simulink model "drivecycle"  (R2024b)
settings: Solver=VariableStepAuto  StartTime=0.0  StopTime=1800  RelTol=1e-3
undefined symbols (not defined in the file or in its folder): Ion, Lithium
libraries: nesl_utility x6, sdl_lib x2, spsBatteryLib x1, autolibmappedmotor x1, fl_lib x1, slpidlib x1, sps_lib x1
settings Model: SimulationMode=accelerator  Creator=srich  LastModifiedBy=srich
settings DataIOCC: LoggingToFile=on

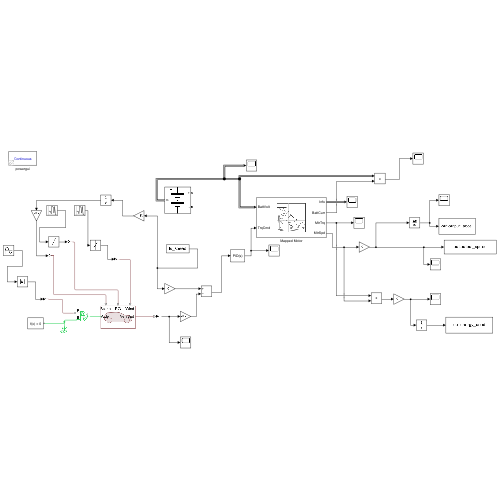
[thumbnail: Simulink's stored preview of the top-level diagram]
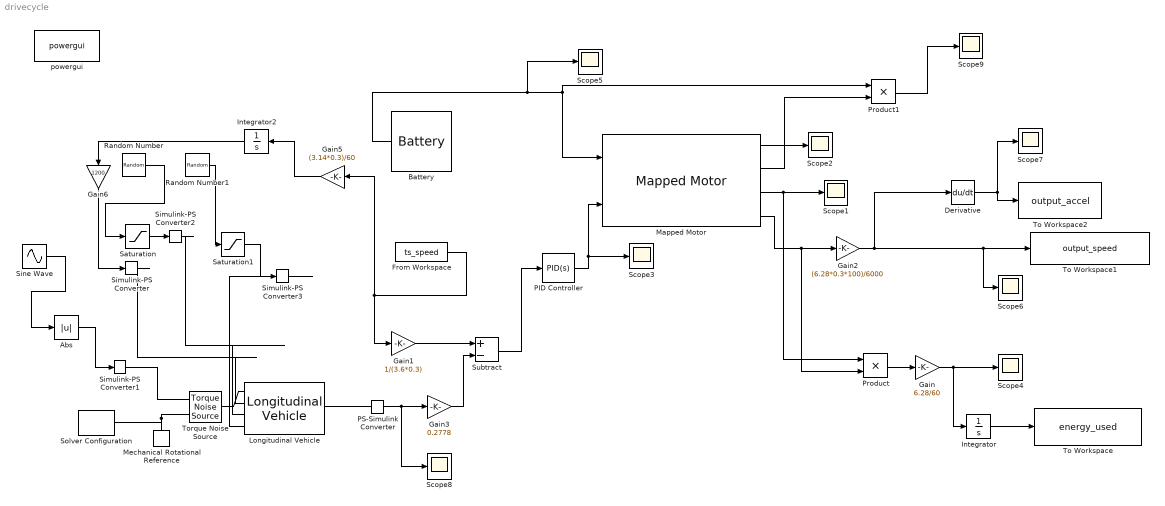
== system drivecycle ==
  Abs : Abs  SaturateOnIntegerOverflow=off
  Battery : spsBatteryLib/Battery  BatType=Lithium-Ion  NomV=360  NomQ=120  SOC=100  Batt_Tr=1e-3  PresetModel=on  MaxQ=120  MinV=270  FullV=419.0354  Dis_rate=52.1739  R=0.03  Normal_OP=108.5217  expZone="[388.9389      5.895652]"
  Derivative : Derivative
  From Workspace : FromWorkspace  VariableName=ts_speed  SampleTime=-1
  Gain : Gain  Gain=6.28/60
  Gain1 : Gain  Gain=1/(3.6*0.3)
  Gain2 : Gain  Gain=(6.28*0.3*100)/6000
  Gain3 : Gain  Gain=0.2778
  Gain5 : Gain  Gain=(3.14*0.3)/60
  Gain6 : Gain  Gain=1200
  Integrator : Integrator
  Integrator2 : Integrator
  Longitudinal Vehicle : sdl_lib/Tires & Vehicles/Longitudinal Vehicle  vehParamType=sdl.enum.VehicleParameterizationType.Regular  M_vehicle=1200 kg  R_tireroll=0.3 m  C_tireroll=0.015  C_airdrag=0.29  A_front=2.2 m^2  A_rl=120 N  B_rl=1.8 N*s/m  C_rl=0.389 N*s^2/m^2  g=9.81 m/s^2  V_1=0.3 m/s  w_1=0.01 rad/s  ShowBrakeIn=true  ShowSlopeIn=true  SlopeInputType=sdl.enum.VehicleLongitudinalRoadSlopeInputType.GradePercent  ShowWindIn=true  ShowGOut=false  air_density=1.184 kg/m^3  V_x_specify=off  V_x_priority=High  V_x=0 m/s  V_x_nominal_specify=off  V_x_nominal_value=1  V_x_nominal_unit=m/s  trq_specify=off  trq_priority=None  trq=0 N*m  trq_nominal_specify=off  trq_nominal_value=1  trq_nominal_unit=N*m  w_specify=off  w_priority=None  w=0 rad/s  w_nominal_specify=off  w_nominal_value=1  w_nominal_unit=rad/s
      settings: InternalSimscapePortConfiguration="{\"Bottom\":[],\"Left\":[{\"id\":\"Axle\",\"label\":\"Axle\",\"type\":\"foundation.mechanical.rotational.rotational\"}],\"Right\":[{\"id\":\"v_out\",\"label\":\"VehSpd\",\"type\":\"output\"}],\"Top\":[{\"id\":\"brkF\",\"label\":\"Brake\",\"type\":\"input\"},{\"id\":\"grade_pct\",\"label\":\"PG\",\"type\":\"input\"},{\"id\":\"V_wind\",\"label\":\"Wind\",\"type\":\"input\"}]}"
  Mapped Motor : autolibmappedmotor/Mapped Motor  w_Tmax_bp_ext=w_Tmax_bp  Tmax_w_V_ext=Tmax_w_V  w_Tmin_bp_ext=w_Tmin_bp  Tmin_w_V_ext=Tmin_w_V  port_config=Torque  param_by=Tabulated torque-speed envelope  w_t=[ 0 375 750 800 ]  T_t=[0.09 0.08 0.07 0]  torque_max=.1  power_max=30  SpreadsheetTqLimitsFileName=MotorCalibrationImportData.xlsx  Tmax_w_V=[0.09 0.09 0.09;0.08 0.08 0.08;0.07 0.07 0.07;0 0 0]  w_Tmax_bp=[ 0 375 750 800 ]  V_Tmax_bp=[500 750 900]  Tmin_w_V=[-0.09 -0.09 -0.09;-0.08 -0.08 -0.08;-0.07 -0.07 -0.07;0 0 0]  w_Tmin_bp=[ 0 375 750 800 ]  V_Tmin_bp=[500 750 900]  Tc=0.02  param_loss=Single efficiency measurement  SpreadsheetLossFileName=MotorCalibrationImportData.xlsx  SpreadsheetEffFileName=MotorCalibrationImportData.xlsx  eff=100  w_eff=375  T_eff=0.08  Piron=0  Pbase=0  w_eff_bp=[-800 -400 0 400 800]  T_eff_bp=[0 0.03 0.06 0.09]  Temp_eff_bp=[233.15 293.15 373.15]  V_eff_bp=[500 700 900]  losses_table=[1.49 1.67 2.21 3.10; 0.42 0.69 1.14 2.03; 0.06 0.24 0.78 1.68; 0.42 0.69 1.14 2.03; 1.49 1.67 2.21 3.10]  losses_table_3d=cat(3,[1.49 1.67 2.21 3.10; 0.42 0.69 1.14 2.03; 0.06 0.24 0.78 1.68; 0.42 0.69 1.14 2.03; 1.49 1.67 2.21 3.10],[1.49 1.67 2.21 3.10; 0.42 0.69 1.14 2.03; 0.06 0.24 0.78 1.68; 0.42 0.69 1.14 2.03; 1.49 1.67 2.21 3.10],[1.49 1.67 2.21 3.10; 0.42 0.69 1.14 2.03; 0.06 0.24 0.78 1.68; 0.42 0.69 1.14 2.03; 1.49 1.67 2.21 3.10])  losses_table_4d=cat(4,cat(3,[1.5645 0.441 0.063 0.441 1.5645;1.7535 0.7245 0.252 0.7245 1.7535;2.3205 1.197 0.819 1.197 2.3205;3.255 2.1315 1.764 2.1315 3.255],[1.5645 0.441 0.063 0.441 1.5645;1.7535 0.7245 0.252 0.7245 1.7535;2.3205 1.197 0.819 1.197 2.3205;3.255 2.1315 1.764 2.1315 3.255],[1.5645 0.441 0.063 0.441 1.5645;1.7535 0.7245 0.252 0.7245 1.7535;2.3205 1.197 0.819 1.197 2.3205;3.255 2.1315 1.764 2.1315 3.255]),cat(3,[1.49 0.42 0.06 0.42 1.49;1.67 0.69 0.24 0.69 1.67;2.21 1.14 0.78 1.14 2.21;3.1 2.03 1.68 2.03 3.1],[1.49 0.42 0.06 0.42 1.49;1.67 0.69 0.24 0.69 1.67;2.21 1.14 0.78 1.14 2.21;3.1 2.03 1.68 2.03 3.1],[1.49 0.42 0.06 0.42 1.49;1.67 0.69 0.24 0.69 1.67;2.21 1.14 0.78 1.14 2.21;3.1 2.03 1.68 2.03 3.1]),cat(3,[1.5347 0.4326 0.0618 0.4326 1.5347;1.7201 0.7107 0.2472 0.7107 1.7201;2.2763 1.1742 0.8034 1.1742 2.2763;3.193 2.0909 1.7304 2.0909 3.193],[1.5347 0.4326 0.0618 0.4326 1.5347;1.7201 0.7107 0.2472 0.7107 1.7201;2.2763 1.1742 0.8034 1.1742 2.2763;3.193 2.0909 1.7304 2.0909 3.193],[1.5347 0.4326 0.0618 0.4326 1.5347;1.7201 0.7107 0.2472 0.7107 1.7201;2.2763 1.1742 0.8034 1.1742 2.2763;3.193 2.0909 1.7304 2.0909 3.193]))  efficiency_table=[95 95 95 95; 95 95 95 95; 95 95 95 95; 95 95 95 95; 95 95 95 95]  efficiency_table_3d=cat(3,[95 95 95 95; 95 95 95 95; 95 95 95 95; 95 95 95 95; 95 95 95 95],[95 95 95 95; 95 95 95 95; 95 95 95 95; 95 95 95 95; 95 95 95 95],[95 95 95 95; 95 95 95 95; 95 95 95 95; 95 95 95 95; 95 95 95 95])  efficiency_table_4d=cat(4,cat(3,90*ones(5,4)',90*ones(5,4)',90*ones(5,4)'),cat(3,95*ones(5,4)',95*ones(5,4)',95*ones(5,4)'),cat(3,92*ones(5,4)',92*ones(5,4)',92*ones(5,4)'))  J=5e-6  b=1e-5  omega_o=0  T_t_extended=[0 0.07 0.08 0.09 0.08 0.07 0]  w_t_extended=[-800 -750 -375 0 375 750 800]  KLossIron=0  KLossCopper=0  x_w_eff_vec=[-8000 -4000 0 4000 8000]  x_T_eff_vec=[-0.09 -0.06 -0.03 0 0.03 0.06 0.09]  x_tmp_eff_vec=[-0.09 -0.06 -0.03 0 0.03 0.06 0.09]  x_V_eff_vec=[500 700 900]  x_losses_mat=[3.1 2.21 1.67 1.49 1.67 2.21 3.1;2.03 1.14 0.69 0.42 0.69 1.14 2.03;1.68 0.78 0.24 0.06 0.24 0.78 1.68;2.03 1.14 0.69 0.42 0.69 1.14 2.03;3.1 2.21 1.67 1.49 1.67 2.21 3.1]  x_losses_mat_3d=[37.8947368421052 25.2631578947368 12.6315789473684 0 12 24 36;18.9473684210526 12.6315789473684 6.3157894736842 0 5.99999999999999 12 18;0 0 0 0 0 0 0;18 12 5.99999999999999 0 6.3157894736842 12.6315789473684 18.9473684210526;36 24 12 0 12.6315789473684 25.2631578947368 37.8947368421052]  x_losses_mat_4d=cat(4,cat(3,[1.5645 0.441 0.063 0.441 1.5645;1.7535 0.7245 0.252 0.7245 1.7535;2.3205 1.197 0.819 1.197 2.3205;3.255 2.1315 1.764 2.1315 3.255],[1.5645 0.441 0.063 0.441 1.5645;1.7535 0.7245 0.252 0.7245 1.7535;2.3205 1.197 0.819 1.197 2.3205;3.255 2.1315 1.764 2.1315 3.255],[1.5645 0.441 0.063 0.441 1.5645;1.7535 0.7245 0.252 0.7245 1.7535;2.3205 1.197 0.819 1.197 2.3205;3.255 2.1315 1.764 2.1315 3.255]),cat(3,[1.49 0.42 0.06 0.42 1.49;1.67 0.69 0.24 0.69 1.67;2.21 1.14 0.78 1.14 2.21;3.1 2.03 1.68 2.03 3.1],[1.49 0.42 0.06 0.42 1.49;1.67 0.69 0.24 0.69 1.67;2.21 1.14 0.78 1.14 2.21;3.1 2.03 1.68 2.03 3.1],[1.49 0.42 0.06 0.42 1.49;1.67 0.69 0.24 0.69 1.67;2.21 1.14 0.78 1.14 2.21;3.1 2.03 1.68 2.03 3.1]),cat(3,[1.5347 0.4326 0.0618 0.4326 1.5347;1.7201 0.7107 0.2472 0.7107 1.7201;2.2763 1.1742 0.8034 1.1742 2.2763;3.193 2.0909 1.7304 2.0909 3.193],[1.5347 0.4326 0.0618 0.4326 1.5347;1.7201 0.7107 0.2472 0.7107 1.7201;2.2763 1.1742 0.8034 1.1742 2.2763;3.193 2.0909 1.7304 2.0909 3.193],[1.5347 0.4326 0.0618 0.4326 1.5347;1.7201 0.7107 0.2472 0.7107 1.7201;2.2763 1.1742 0.8034 1.1742 2.2763;3.193 2.0909 1.7304 2.0909 3.193]))  CalLossMapData={}  CalLossWithTempMapData={}  aMode=1  RefBlkName='autolibmappedmotor/Mapped Motor'
      settings: LibrarySourceBlock=autolibemachines/Mapped Motor
  Mechanical Rotational Reference : fl_lib/Mechanical/Rotational Elements/Mechanical Rotational Reference
  PID Controller : slpidlib/PID Controller  Controller=PID  Form=Parallel  TimeDomain=Continuous-time  UseExternalTs=off  SampleTime=-1  IntegratorMethod=Forward Euler  FilterMethod=Forward Euler  ControllerParametersSource=internal  P=1  I=0.1  UseKiTs=off  D=0.01  UseExternalDerivativeSource=off  N=1  UseFilter=on  TunerSelectOption=Transfer Function Based (PID Tuner App)  InitialConditionSource=internal  InitialConditionForIntegrator=0  InitialConditionForFilter=0  DifferentiatorICPrevScaledInput=0  ExternalReset=none  TrackingMode=off  Kt=1  LimitOutput=off  SatLimitsSource=internal  UpperSaturationLimit=inf  LowerSaturationLimit=-inf  LinearizeAsGain=on  AntiWindupMode=none  Kb=1  LimitIntegrator=off  UpperIntegratorSaturationLimit=inf  LowerIntegratorSaturationLimit=-inf  POutMin=[]  POutMax=[]  IOutMin=[]  IOutMax=[]  DOutMin=[]  DOutMax=[]  NOutMin=[]  NOutMax=[]  SumOutMin=[]  SumOutMax=[]  SaturationOutMin=[]  SaturationOutMax=[]  PParamMin=[]  PParamMax=[]  IParamMin=[]  IParamMax=[]  DParamMin=[]  DParamMax=[]  NParamMin=[]  NParamMax=[]  KbParamMin=[]  KbParamMax=[]  KtParamMin=[]  KtParamMax=[]  KbOutMin=[]  KbOutMax=[]  KtOutMin=[]  KtOutMax=[]  IntegratorOutMin=[]  IntegratorOutMax=[]  FilterOutMin=[]  FilterOutMax=[]  SumI1OutMin=[]  SumI1OutMax=[]  SumI2OutMin=[]  SumI2OutMax=[]  SumI3OutMin=[]  SumI3OutMax=[]  SumI4OutMin=[]  SumI4OutMax=[]  SumDOutMin=[]  SumDOutMax=[]  DifferentiatorOutMin=[]  DifferentiatorOutMax=[]  FilterDiffOutCoefMin=[]  FilterDiffOutCoefMax=[]  ReciprocalOutMin=[]  ReciprocalOutMax=[]  SumDenOutMin=[]  SumDenOutMax=[]  SumNumOutMin=[]  SumNumOutMax=[]  DivideOutMin=[]  DivideOutMax=[]  UdiffTsProdOutMin=[]  UdiffTsProdOutMax=[]  NTsProdOutMin=[]  NTsProdOutMax=[]  UintegralTsProdOutMin=[]  UintegralTsProdOutMax=[]  UngainTsProdOutMin=[]  UngainTsProdOutMax=[]  ClampingZeroOutDataTypeStr=Inherit: Inherit via back propagation  ClampingZeroOutMin=[]  ClampingZeroOutMax=[]  FilterDenConstantOutDataTypeStr=Inherit: Inherit via back propagation  FilterDenConstantOutMin=[]  FilterDenConstantOutMax=[]  PCopyOutDataTypeStr=Inherit: Inherit via back propagation  PCopyOutMin=[]  PCopyOutMax=[]  NCopyOutDataTypeStr=Inherit: Inherit via back propagation  NCopyOutMin=[]  NCopyOutMax=[]  IntegratorContinuousStateAttributes=''  IntegratorStateMustResolveToSignalObject=off  IntegratorRTWStateStorageClass=Auto  FilterContinuousStateAttributes=''  FilterStateMustResolveToSignalObject=off  FilterRTWStateStorageClass=Auto  ParallelPVariant=InternalParameters  IdealPVariant=Disabled  IVariant=InternalParameters  DVariant=InternalParameters  IntegratorVariant=Continuous  SatVariant=Disabled  AWVariant=Passthrough  PCopyVariant=Disabled  TRVariant=Disabled  FdbkBlocksVariant=Forward  IdealPFdbkVariant=Disabled  SatFdbkVariant=Disabled  DerivativeFilterVariant=ContFilter  NVariant=InternalParameters  NCopyVariant=Disabled  FilterICVariant=InternalICsFilter  IntegratorICVariant=InternalICs  ExternalResetVariant=Disabled  TRSumVariant=Passthrough  SumFdbkVariant=Disabled  SumVariant=Sum_PID  TsampFilterVariant=InternalTs  TsampNgainVariant=Passthrough  TsampIntegralVariant=Disabled_SignalSpec  ExternalSaturationOutDataTypeStr=Inherit: Same as second input  DerivativeSourceVariant=ErrorSignal  PreIntVariant=InternalPreInt
  PS-Simulink Converter : nesl_utility/PS-Simulink Converter  PhysicalDomain=network_engine_domain  SubClassName=ps_output  LeftPortType=input  RightPortType=output  PseudoPeriodic=off  Frequencies=[]  VectorFormat=inherit  Unit=inherit  AffineConversion=off
  Product : Product
  Product1 : Product
  Random Number : RandomNumber  Mean=6.5  Variance=0.5625  SampleTime=0.01
  Random Number1 : RandomNumber  Mean=7.5  Variance=0.5625  SampleTime=0.1
  Saturation : Saturate  UpperLimit=8  LowerLimit=5
  Saturation1 : Saturate  UpperLimit=10  LowerLimit=5
  Scope{1..9} (9 alike) : Scope
  Simulink-PS Converter{,1..3} (4 alike) : nesl_utility/Simulink-PS Converter  PhysicalDomain=network_engine_domain  SubClassName=ps_input  LeftPortType=input  RightPortType=output  PseudoPeriodic=off  Frequencies=[]  NoiseDistribution=none  NoiseParameters=[]  Unit=1  AffineConversion=off  FilteringAndDerivatives=provide  SimscapeFilterOrder=1  InputFilterTimeConstant=0.001  UdotUserProvided=0
  Sine Wave : Sin  Amplitude=5  Bias=5  Frequency=10  SampleTime=0
  Solver Configuration : nesl_utility/Solver Configuration  PhysicalDomain=network_engine_domain  SubClassName=solver  LeftPortType=input  RightPortType=generic  Tones=[]  Harmonics=[]  SimulateNoise=off  Profile=off  UseLocalSampling=off  EnableSwitchedLinearOptims=on  FrequencyDomain=off  UseCCode=off  RelTol=0.001  AbsTol=0.001  MinStep=1e-09  ToWorkspace=off  RevertToSquareIcSolve=off  NumHomotopyIterations=100  PhasorMode=off  PhasorModeNumHarmonics=1  ConsistencySolver=NEWTON_XTOL_AFTER_FTOL  IndexReductionMethod=DerivativeReplacement  DoDC=off  ResidualTolerance=1e-09  ConsistencyTolSource=GLOBAL  ConsistencyAbsTol=0.001  ConsistencyRelTol=0.001  ConsistencyTolFactor=0.001  UseLocalSolver=off  LocalSolverChoice=NE_BACKWARD_EULER_ADVANCER  ResolveIndetEquations=on  FunctionEvalNumThread=1  LocalSolverSampleTime=0.001  DoFixedCost=off  MaxNonlinIter=3  MaxModeIter=2  ComputeImpulses=off  ImpulseIterations=2  LinearAlgebra=auto  LinearAlgebraNumThread=0  EquationFormulation=NE_TIME_EF  DelaysMemoryBudget=1024  AutomaticFiltering=on  FilteringTimeConstant=0.001  PartitionStorageMethod=AS_NEEDED  PartitionMemoryBudget=1024  PartitionMethod=ROBUST  MultibodyUseLocalSolver=off  MultibodyLocalSolverChoice=ODE1  MultibodyLocalSolverSampleTime=0.001
  Subtract : Sum  Inputs=+-
  To Workspace : ToWorkspace  VariableName=energy_used  SaveFormat=Timeseries
  To Workspace1 : ToWorkspace  VariableName=output_speed  SaveFormat=Timeseries
  To Workspace2 : ToWorkspace  VariableName=output_accel  SaveFormat=Timeseries
  Torque Noise Source : sdl_lib/Sources/Torque Noise Source  sample_time=1e-3 s  repeatability=sdl.enum.seedInitialization.NotRepeatable  user_seed=0  auto_seed=3890346746
      settings: InternalSimscapePortConfiguration="{\"Bottom\":[],\"Left\":[{\"id\":\"PSD\",\"label\":\"P\",\"type\":\"input\"},{\"id\":\"B\",\"label\":\"B\",\"type\":\"foundation.mechanical.rotational.rotational\"}],\"Right\":[{\"id\":\"F\",\"label\":\"F\",\"type\":\"foundation.mechanical.rotational.rotational\"}],\"Top\":[]}"
  powergui : sps_lib/powergui  Priority=1  SimulationMode=Continuous  SampleTime=1800  frequency=60  Iterations=50  frequencyindice=0  Pbase=100e6  ErrMax=1e-4  UnitsV=kV  UnitsW=MW  buscounter=0  FunctionMessages=off  echomessages=off  EnableUseOfTLC=off  CurrentSourceSwitches=off  DisableSnubberDevices=off  DisableRonSwitches=off  DisableVfSwitches=off  DisplayEquations=off  AutomaticDiscreteSolvers=off  SolverType=Tustin/Backward Euler (TBE)  Interpol=off  ExternalGateDelay=off  methode=off  Ts=100  x0status=blocks  SPID=on  SwTol=0  HookPort=off  NonlinearTolerance=1e-4  nMaxIteration=100  ContinueOnMaxIteration=off  RestoreLinks=warning  ResistiveCurrentMeasurement=off  Frange=[0:2:500]  Ylog=off  Xlog=on  ShowGrid=off  save=off  variable=ZData  structure=0  ZoomFFT=off  StartTime=0.0  cycles=1  DisplayStyle=1  fundamental=60  FreqAxis=off  MaxFrequency=1000  frequencyindicesteady=1  RmsSteady=1  display=off
  wires:
  Derivative/1 -> Scope7/1, To Workspace2/1
  From Workspace/1 -> Gain1/1, Gain5/1
  Battery/1 -> Scope5/1, Mapped Motor/1, Product1/1
  PID Controller/1 -> Mapped Motor/2, Scope3/1
  Gain1/1 -> Subtract/1
  PS-Simulink Converter/1 -> Scope8/1, Gain3/1
  Gain3/1 -> Subtract/2
  Subtract/1 -> PID Controller/1
  Sine Wave/1 -> Abs/1
  Abs/1 -> Simulink-PS Converter1/1
  Mapped Motor/3 -> Product/1, Scope1/1
  Mapped Motor/1 -> Scope2/1
  Mapped Motor/4 -> Gain2/1, Product/2
  Gain2/1 -> Derivative/1, Scope6/1, To Workspace1/1
  Gain5/1 -> Integrator2/1
  Integrator2/1 -> Gain6/1
  Gain6/1 -> Simulink-PS Converter/1
  Random Number/1 -> Saturation/1
  Saturation/1 -> Simulink-PS Converter2/1
  Saturation1/1 -> Simulink-PS Converter3/1
  Random Number1/1 -> Saturation1/1
  Product/1 -> Gain/1
  Gain/1 -> Scope4/1, Integrator/1
  Integrator/1 -> To Workspace/1
  Mapped Motor/2 -> Product1/2
  Product1/1 -> Scope9/1
  connections:
  PS-Simulink Converter/LConn1 -- Longitudinal Vehicle/RConn1
  Torque Noise Source/RConn1 -- Longitudinal Vehicle/LConn1
  Simulink-PS Converter1/RConn1 -- Torque Noise Source/LConn1
  Mechanical Rotational Reference/LConn1 -- Solver Configuration/RConn1 -- Torque Noise Source/LConn2
  Simulink-PS Converter/RConn1 -- Longitudinal Vehicle/LConn2
  Simulink-PS Converter2/RConn1 -- Longitudinal Vehicle/LConn3
  Simulink-PS Converter3/RConn1 -- Longitudinal Vehicle/LConn4
